simulink model "Buck_Converter_with_3ph_Full_Bridge_Rectifier"  (R2022b)
settings: Solver=VariableStepAuto  StartTime=0.0  StopTime=.1  RelTol=1e-3
libraries: spsDiodeLib x7, spsSeriesRLCBranchLib x6, spsVoltageMeasurementLib x5, spsGroundLib x4, spsDCVoltageSourceLib x3, spsCurrentMeasurementLib x1, spsDCMachineLib x1, spsIGBTLib x1, spsThreePhaseVIMeasurementLib x1, spsThreePhaseSourceLib x1, spspowerguiLib x1
settings Model: Creator=meteh  LastModifiedBy=meteh
settings SolverCC: ZeroCrossAlgorithm=Adaptive
settings DebuggingCC: IgnoredZcDiagnostic=none

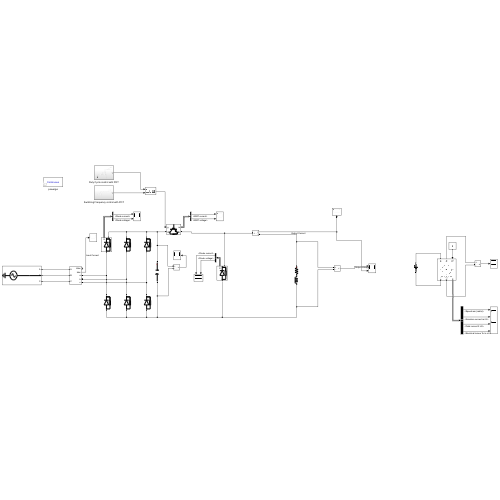
[thumbnail: Simulink's stored preview of the top-level diagram]
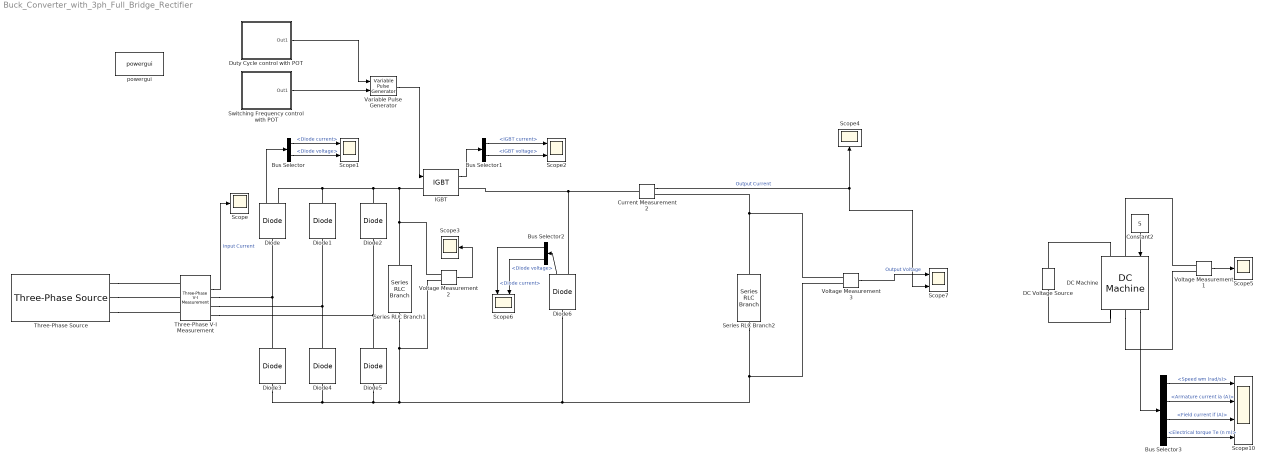
== system Buck_Converter_with_3ph_Full_Bridge_Rectifier ==
  Bus Selector : BusSelector  OutputSignals=Diode current,Diode voltage
  Bus Selector1 : BusSelector  OutputSignals=IGBT current,IGBT voltage
  Bus Selector2 : BusSelector  OutputSignals=Diode current,Diode voltage
  Bus Selector3 : BusSelector  OutputSignals=Speed wm (rad/s),Armature current ia (A),Field current if (A),Electrical torque Te (n m)
  Constant2 : Constant  Value=5
  Current Measurement2 : spsCurrentMeasurementLib/Current Measurement  PhasorSimulation=off  OutputType=Complex  PSBequivalent=0
  DC Machine : spsDCMachineLib/DC Machine  PresetModel=No  MechanicalLoad=Torque TL  FieldType=Wound  ShowDetailedParameters=on  MeasurementBus=off  RLa="[ 0.8  0.0125]"  RLf="[ 210  23]"  Laf=1  MachineConstant=Torque constant (N.m/A)  Ke=1.8  Kt=1.8  J=0.5  Bm=0  Tf=0  w0=0  Ifinit=1.04761904761905  TsPowergui=0  TsBlock=-1
  DC Voltage Source : spsDCVoltageSourceLib/DC Voltage Source  Amplitude=220  Measurements=None
  Diode : spsDiodeLib/Diode  Ron=0.001  Lon=0  Vf=0.8  IC=0  UseSnubber=0  Rs=500  Cs=250e-9  Measurements=on
  Diode{1..5} (5 alike) : spsDiodeLib/Diode  Ron=0.001  Lon=0  Vf=0.8  IC=0  UseSnubber=0  Rs=500  Cs=250e-9  Measurements=off
  Diode6 : spsDiodeLib/Diode  Ron=0.001  Lon=0  Vf=0.8  IC=0  UseSnubber=0  Rs=500  Cs=250e-9  Measurements=on
  Duty Cycle control with POT : Subsystem
  IGBT : spsIGBTLib/IGBT  Ron=0.001  Lon=0  Vf=1  Tf=1e-6  Tt=2e-6  IC=0  Rs=1e5  Cs=1e-9  Measurements=on
  Scope{,3..5} (4 alike) : Scope
  Scope{1..2,6..7} (4 alike) : Scope  NumInputPorts=2
  Scope10 : Scope  NumInputPorts=4
  Series RLC Branch1 : spsSeriesRLCBranchLib/Series RLC Branch  LConnTagsString=__new0  RConnTagsString=__new0  BranchType=C  Resistance=0.8  Inductance=12.5e-3  SetiL0=off  InitialCurrent=0  Capacitance=1410e-6  Setx0=off  InitialVoltage=0  Measurements=None
  Series RLC Branch2 : spsSeriesRLCBranchLib/Series RLC Branch  LConnTagsString=__new0  RConnTagsString=__new0  BranchType=RL  Resistance=0.8  Inductance=12.5e-3  SetiL0=off  InitialCurrent=0  Capacitance=1410e-6  Setx0=off  InitialVoltage=0  Measurements=None
  Switching Frequency control with POT : Subsystem
  Three-Phase V-I Measurement : spsThreePhaseVIMeasurementLib/Three-Phase V-I Measurement  VoltageMeasurement=phase-to-ground  SetLabelV=off  LabelV=Vabc  Vpu=off  VpuLL=off  CurrentMeasurement=yes  SetLabelI=off  LabelI=Iabc  Ipu=off  Pbase=100e6  Vbase=500e3  OutputType=Complex  PhasorSimulation=off  PSBequivalent=0
  Three-Phase Source : spsThreePhaseSourceLib/Three-Phase Source  InternalConnection=Yg  VoltagePhases=off  Voltage=140  PhaseAngle=0  Voltage_phases=[25e3 25e3 25e3]/sqrt(3)  PhaseAngles_phases=[0 -120 +120]  Frequency=50  NonIdealSource=off  SpecifyImpedance=off  Resistance=0.008929  Inductance=1.658e-3  ShortCircuitLevel=100e6  BaseVoltage=25e3  XRratio=7  BusType=swing  Pref=10e3  Qref=0  Prefabc=[10e3, 10e3, 10e3]  Qrefabc=[0, 0, 0]  Qmin=-inf  Qmax=inf
  Variable Pulse Generator : VariablePulseGenerator  SampleTime=0.1
  Voltage Measurement1 : spsVoltageMeasurementLib/Voltage Measurement  PhasorSimulation=off  OutputType=Complex  PSBequivalent=0
  Voltage Measurement2 : spsVoltageMeasurementLib/Voltage Measurement  PhasorSimulation=off  OutputType=Complex  PSBequivalent=0
  Voltage Measurement3 : spsVoltageMeasurementLib/Voltage Measurement  PhasorSimulation=off  OutputType=Complex  PSBequivalent=0
  powergui : spspowerguiLib/powergui  Priority=1  SimulationMode=Continuous  SampleTime=50e-6  frequency=60  Iterations=50  frequencyindice=0  Pbase=100e6  ErrMax=1e-4  UnitsV=kV  UnitsW=MW  buscounter=0  FunctionMessages=off  echomessages=off  EnableUseOfTLC=off  CurrentSourceSwitches=off  DisableSnubberDevices=off  DisableRonSwitches=off  DisableVfSwitches=off  DisplayEquations=off  AutomaticDiscreteSolvers=off  SolverType=Tustin/Backward Euler (TBE)  Interpol=off  ExternalGateDelay=off  methode=off  Ts=100  x0status=blocks  SPID=on  SwTol=0  HookPort=off  NonlinearTolerance=1e-4  nMaxIteration=100  ContinueOnMaxIteration=off  RestoreLinks=warning  ResistiveCurrentMeasurement=off  Frange=[0:2:500]  Ylog=off  Xlog=on  ShowGrid=off  save=off  variable=ZData  structure=0  ZoomFFT=off  StartTime=0.0  cycles=1  DisplayStyle=1  fundamental=60  FreqAxis=off  MaxFrequency=1000  frequencyindicesteady=1  RmsSteady=1  display=off
  wires:
  Diode/1 -> Bus Selector/1
  Bus Selector/1 -> Scope1/1  "<Diode current>"
  Bus Selector/2 -> Scope1/2  "<Diode voltage>"
  Voltage Measurement1/1 -> Scope5/1
  Constant2/1 -> DC Machine/1
  DC Machine/1 -> Bus Selector3/1
  Bus Selector3/1 -> Scope10/1  "<Speed wm (rad/s)>"
  Bus Selector3/2 -> Scope10/2  "<Armature current ia (A)>"
  Bus Selector3/3 -> Scope10/3  "<Field current if (A)>"
  Bus Selector3/4 -> Scope10/4  "<Electrical torque Te (n m)>"
  Three-Phase V-I Measurement/2 -> Scope/1  "Input Current"
  Bus Selector1/1 -> Scope2/1  "<IGBT current>"
  Bus Selector1/2 -> Scope2/2  "<IGBT voltage>"
  IGBT/1 -> Bus Selector1/1
  Current Measurement2/1 -> Scope7/2, Scope4/1  "Output Current"
  Voltage Measurement2/1 -> Scope3/1
  Variable Pulse Generator/1 -> IGBT/1
  Duty Cycle control with POT/1(Out1) -> Variable Pulse Generator/1
  Switching Frequency control with POT/1(Out1) -> Variable Pulse Generator/2
  Bus Selector2/2 -> Scope6/2  "<Diode voltage>"
  Bus Selector2/1 -> Scope6/1  "<Diode current>"
  Diode6/1 -> Bus Selector2/1
  Voltage Measurement3/1 -> Scope7/1  "Output Voltage"
  connections:
  Diode3/RConn1 -- Diode/LConn1 -- Three-Phase V-I Measurement/RConn1
  Diode4/RConn1 -- Three-Phase V-I Measurement/RConn2 -- Diode1/LConn1
  Diode5/RConn1 -- Diode2/LConn1 -- Three-Phase V-I Measurement/RConn3
  Voltage Measurement2/LConn2 -- Series RLC Branch2/RConn1 -- Voltage Measurement3/LConn2 -- Diode6/LConn1 -- Diode3/LConn1 -- Diode4/LConn1 -- Diode5/LConn1 -- Series RLC Branch1/RConn1
  Three-Phase Source/RConn1 -- Three-Phase V-I Measurement/LConn1
  Three-Phase Source/RConn2 -- Three-Phase V-I Measurement/LConn2
  Three-Phase Source/RConn3 -- Three-Phase V-I Measurement/LConn3
  Series RLC Branch1/LConn1 -- Voltage Measurement2/LConn1 -- IGBT/LConn1 -- Diode2/RConn1 -- Diode/RConn1 -- Diode1/RConn1
  Diode6/RConn1 -- IGBT/RConn1 -- Current Measurement2/LConn1
  DC Voltage Source/RConn1 -- DC Machine/LConn2
  DC Machine/RConn2 -- DC Voltage Source/LConn1
  Voltage Measurement1/LConn1 -- DC Machine/LConn1
  DC Machine/RConn1 -- Voltage Measurement1/LConn2
  Series RLC Branch2/LConn1 -- Voltage Measurement3/LConn1 -- Current Measurement2/RConn1

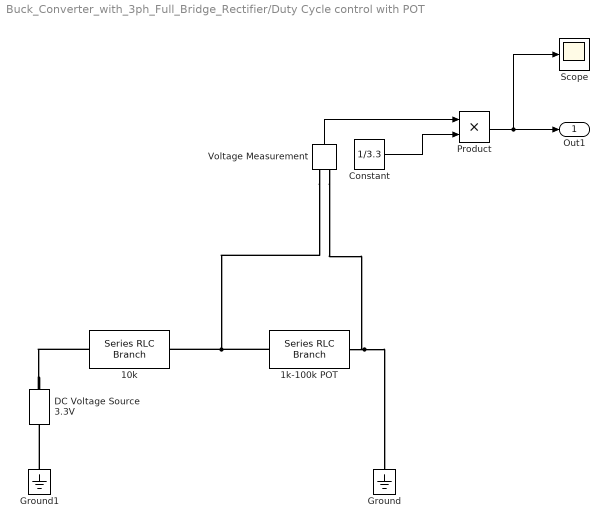
== system Buck_Converter_with_3ph_Full_Bridge_Rectifier/Duty Cycle control with POT ==
  "10k " : spsSeriesRLCBranchLib/Series RLC Branch  LConnTagsString=__new0  RConnTagsString=__new0  BranchType=R  Resistance=1e4  Inductance=1e-3  SetiL0=off  InitialCurrent=0  Capacitance=1e-6  Setx0=off  InitialVoltage=0  Measurements=None
  1k-100k POT : spsSeriesRLCBranchLib/Series RLC Branch  LConnTagsString=__new0  RConnTagsString=__new0  BranchType=R  Resistance=2.5e3  Inductance=1e-3  SetiL0=off  InitialCurrent=0  Capacitance=1e-6  Setx0=off  InitialVoltage=0  Measurements=None
  Constant : Constant  Value=1/3.3
  DC Voltage Source 3.3V : spsDCVoltageSourceLib/DC Voltage Source  Amplitude=3.3  Measurements=None
  Ground : spsGroundLib/Ground  LConnTagsString=a
  Ground1 : spsGroundLib/Ground  LConnTagsString=a
  Product : Product
  Scope : Scope
  Voltage Measurement : spsVoltageMeasurementLib/Voltage Measurement  PhasorSimulation=off  OutputType=Complex  PSBequivalent=0
  Out1 : Outport
  wires:
  Voltage Measurement/1 -> Product/1
  Constant/1 -> Product/2
  Product/1 -> Scope/1, Out1/1
  connections:
  1k-100k POT/RConn1 -- Ground/LConn1 -- Voltage Measurement/LConn2
  1k-100k POT/LConn1 -- Voltage Measurement/LConn1 -- "10k "/RConn1
  "10k "/LConn1 -- DC Voltage Source 3.3V/RConn1
  Ground1/LConn1 -- DC Voltage Source 3.3V/LConn1

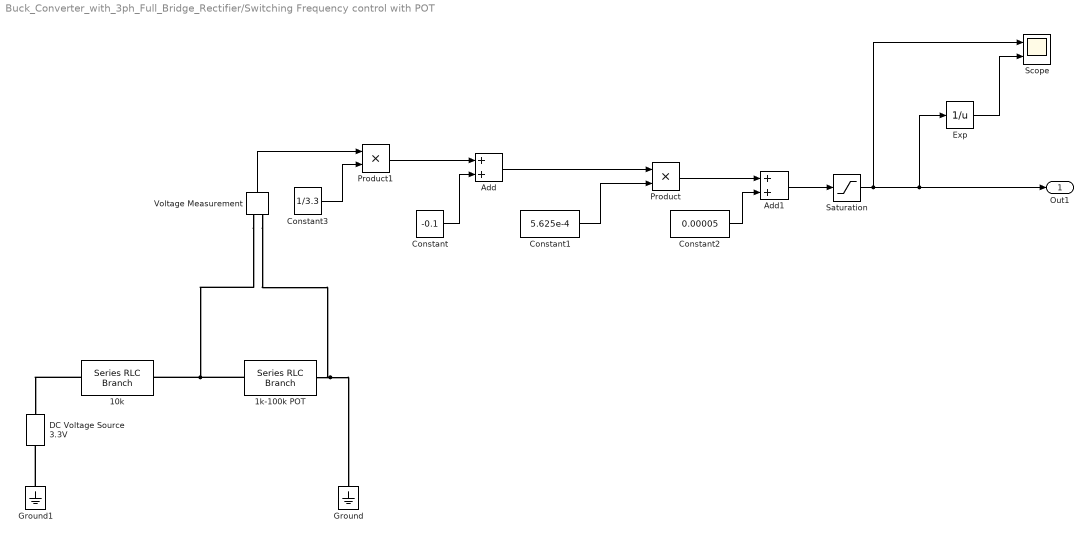
== system Buck_Converter_with_3ph_Full_Bridge_Rectifier/Switching Frequency control with POT ==
  "10k " : spsSeriesRLCBranchLib/Series RLC Branch  LConnTagsString=__new0  RConnTagsString=__new0  BranchType=R  Resistance=1e4  Inductance=1e-3  SetiL0=off  InitialCurrent=0  Capacitance=1e-6  Setx0=off  InitialVoltage=0  Measurements=None
  1k-100k POT : spsSeriesRLCBranchLib/Series RLC Branch  LConnTagsString=__new0  RConnTagsString=__new0  BranchType=R  Resistance=2.5e3  Inductance=1e-3  SetiL0=off  InitialCurrent=0  Capacitance=1e-6  Setx0=off  InitialVoltage=0  Measurements=None
  Add : Sum
  Add1 : Sum
  Constant : Constant  Value=-0.1
  Constant1 : Constant  Value=5.625e-4
  Constant2 : Constant  Value=0.00005
  Constant3 : Constant  Value=1/3.3
  DC Voltage Source 3.3V : spsDCVoltageSourceLib/DC Voltage Source  Amplitude=3.3  Measurements=None
  Exp : Math  Operator=reciprocal
  Ground : spsGroundLib/Ground  LConnTagsString=a
  Ground1 : spsGroundLib/Ground  LConnTagsString=a
  Product : Product
  Product1 : Product
  Saturation : Saturate  UpperLimit=0.001  LowerLimit=0.0001
  Scope : Scope  NumInputPorts=2
  Voltage Measurement : spsVoltageMeasurementLib/Voltage Measurement  PhasorSimulation=off  OutputType=Complex  PSBequivalent=0
  Out1 : Outport
  wires:
  Constant/1 -> Add/2
  Add/1 -> Product/1
  Constant1/1 -> Product/2
  Product/1 -> Add1/1
  Constant2/1 -> Add1/2
  Add1/1 -> Saturation/1
  Saturation/1 -> Scope/1, Exp/1, Out1/1
  Exp/1 -> Scope/2
  Product1/1 -> Add/1
  Voltage Measurement/1 -> Product1/1
  Constant3/1 -> Product1/2
  connections:
  Voltage Measurement/LConn2 -- 1k-100k POT/RConn1 -- Ground/LConn1
  1k-100k POT/LConn1 -- Voltage Measurement/LConn1 -- "10k "/RConn1
  "10k "/LConn1 -- DC Voltage Source 3.3V/RConn1
  Ground1/LConn1 -- DC Voltage Source 3.3V/LConn1
